simulink model "spectrum"  (R2021a)
settings: Solver=VariableStepAuto  StartTime=0.0  StopTime=10.0  RelTol=1e-3
undefined symbols (not defined in the file): Fc, Fm, M
settings Model: Creator=prakh  LastModifiedBy=prakh

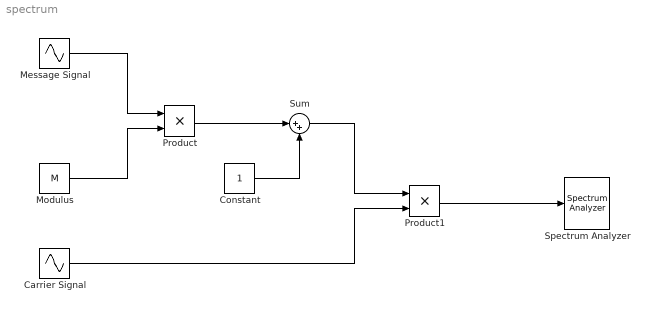
== system spectrum ==
  Carrier Signal : Sin  Frequency=2*pi*Fc  SampleTime=1/1500
  Constant : Constant
  Message Signal : Sin  Frequency=2*pi*Fm  SampleTime=1/1500
  Modulus : Constant  Value=M
  Product : Product
  Product1 : Product
  Spectrum Analyzer : SpectrumAnalyzer
  Sum : Sum  Inputs=|++
  wires:
  Modulus/1 -> Product/2
  Constant/1 -> Sum/2
  Sum/1 -> Product1/1
  Carrier Signal/1 -> Product1/2
  Product/1 -> Sum/1
  Message Signal/1 -> Product/1
  Product1/1 -> Spectrum Analyzer/1
